simulink model "lassistantpeteuncable"  (R2020a)
settings: Solver=VariableStepAuto  StartTime=0.0  StopTime=10.0  RelTol=1e-3
libraries: simulink x2
settings Model: Creator=lab02  LastModifiedBy=lab02

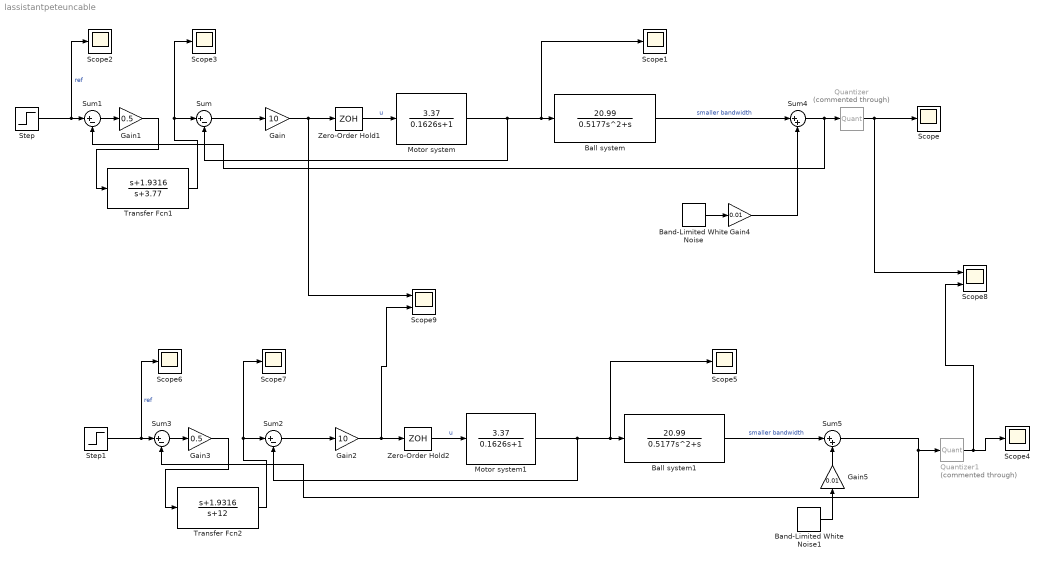
== system lassistantpeteuncable ==
  " Ball system" : TransferFcn  Numerator=[ 20.99]  Denominator=[0.5177 1 0]
  " Ball system1" : TransferFcn  Numerator=[ 20.99]  Denominator=[0.5177 1 0]
  Band-Limited White Noise : simulink/Sources/Band-Limited White Noise  Cov=[5]  Ts=0.1  seed=[23341]
  Band-Limited White Noise1 : simulink/Sources/Band-Limited White Noise  Cov=[5]  Ts=0.1  seed=[23341]
  Gain : Gain  Gain=10
  Gain1 : Gain  Gain=0.5
  Gain2 : Gain  Gain=10
  Gain3 : Gain  Gain=0.5
  Gain4 : Gain  Gain=0.01
  Gain5 : Gain  Gain=0.01
  Motor system : TransferFcn  Numerator=[0 3.37]  Denominator=[0.1626 1]
  Motor system1 : TransferFcn  Numerator=[0 3.37]  Denominator=[0.1626 1]
  Quantizer : Quantizer  Commented=through
  Quantizer1 : Quantizer  Commented=through
  Scope{,1..7} (8 alike) : Scope
  Scope8 : Scope  NumInputPorts=2
  Scope9 : Scope  NumInputPorts=2
  Step : Step
  Step1 : Step
  Sum{,1..3} (4 alike) : Sum  Inputs=|+-
  Sum4 : Sum  Inputs=|++
  Sum5 : Sum  Inputs=|++
  Transfer Fcn1 : TransferFcn  Numerator=[1 1.9316]  Denominator=[1 3.77]
  Transfer Fcn2 : TransferFcn  Numerator=[1 1.9316]  Denominator=[1 12]
  Zero-Order Hold1 : ZeroOrderHold  SampleTime=0.005
  Zero-Order Hold2 : ZeroOrderHold  SampleTime=0.005
  wires:
  Gain5/1 -> Sum5/2
  Gain4/1 -> Sum4/2
  Band-Limited White Noise1/1 -> Gain5/1
  Sum4/1 -> Sum1/2, Quantizer/1
  Quantizer1/1 -> Scope8/2, Scope4/1
  Band-Limited White Noise/1 -> Gain4/1
  Gain2/1 -> Scope9/2, Zero-Order Hold2/1
  Motor system1/1 -> Sum2/2, Scope5/1, " Ball system1"/1
  Zero-Order Hold2/1 -> Motor system1/1  "u"
  Sum3/1 -> Gain3/1
  " Ball system1"/1 -> Sum5/1  "smaller bandwidth"
  Sum5/1 -> Sum3/2, Quantizer1/1
  Gain3/1 -> Transfer Fcn2/1
  Quantizer/1 -> Scope8/1, Scope/1
  Transfer Fcn2/1 -> Sum2/1, Scope7/1
  Step1/1 -> Scope6/1, Sum3/1  "ref"
  Step/1 -> Scope2/1, Sum1/1  "ref"
  Sum2/1 -> Gain2/1
  Gain1/1 -> Transfer Fcn1/1
  Transfer Fcn1/1 -> Sum/1, Scope3/1
  Sum1/1 -> Gain1/1
  " Ball system"/1 -> Sum4/1  "smaller bandwidth"
  Sum/1 -> Gain/1
  Zero-Order Hold1/1 -> Motor system/1  "u"
  Motor system/1 -> Sum/2, Scope1/1, " Ball system"/1
  Gain/1 -> Scope9/1, Zero-Order Hold1/1
